simulink library "component_lib"  (R2023a)
settings: Solver=VariableStepAuto  StartTime=0.0  StopTime=10.0  RelTol=1e-3
undefined symbols (not defined in the file or in its folder): ECCV_r, par, R1234yf_ph, V_nom
libraries: base_lib x258, $bdroot x212, simulink x2, slpidlib x1
(part 7 of 7)

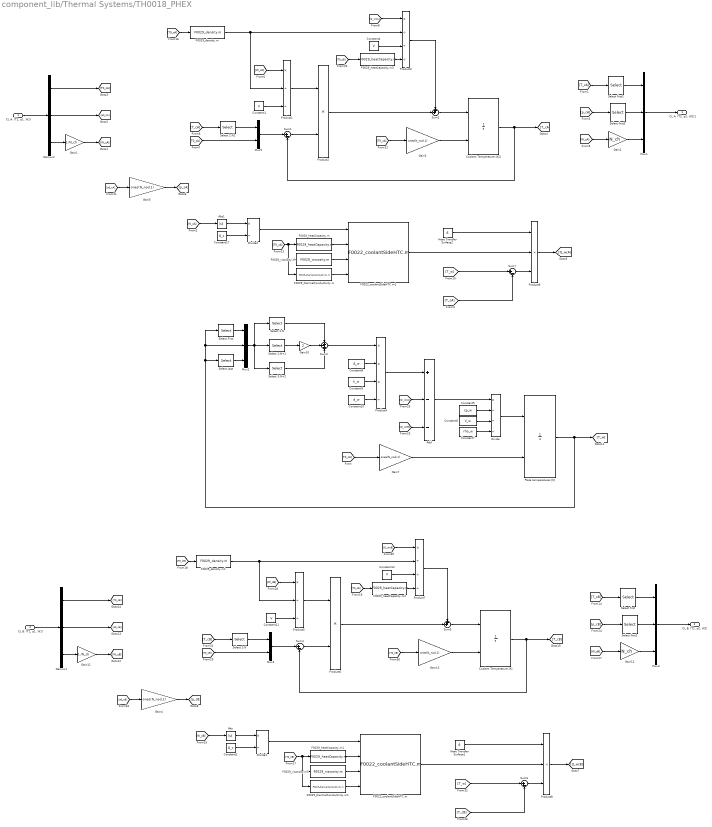
== system component_lib/Thermal Systems/TH0018_PHEX ==
  "CL A: (T1, p1, W1)" : Inport
  "CL B: (T1, p1, W1)" : Inport  Port=2
  Abs : Abs  SaturateOnIntegerOverflow=off
  Abs1 : Abs  SaturateOnIntegerOverflow=off
  Add : Sum  Inputs=+--
  Constant{1,4,11..12} (4 alike) : Constant  Value=V
  Constant10 : Constant  Value=d_w
  Constant17 : Constant  Value=A_c
  Constant2 : Constant  Value=A_c
  Constant5 : Constant  Value=cp_w
  Constant6 : Constant  Value=V_w
  Constant7 : Constant  Value=rho_w
  Constant8 : Constant  Value=A_w
  Constant9 : Constant  Value=k_w
  Coolant Temperature [K] : Integrator  InitialConditionSource=external  LimitOutput=on  LowerSaturationLimit=0
  Coolant Temperature [K]1 : Integrator  InitialConditionSource=external  LimitOutput=on  LowerSaturationLimit=0
  Demux1 : Demux  Outputs=3
  Demux2 : Demux  Outputs=3
  Divide : Product  Inputs=*///
  Divide1 : Product  Inputs=*/
  Divide2 : Product  Inputs=*/
  F0022_coolantSideHTC.m : base_lib/F0022_heatPump/F0022_coolantSideHTC.m  SystemSampleTime=-1  VariantActivationTime=update diagram  Latency=0  AutoFrameSizeCalculation=off
      settings: LibrarySourceBlock=|
      | simulink/User-Defined
      | Functions/MATLAB Function
  F0022_coolantSideHTC.m1 : base_lib/F0022_heatPump/F0022_coolantSideHTC.m  SystemSampleTime=-1  VariantActivationTime=update diagram  Latency=0  AutoFrameSizeCalculation=off
      settings: LibrarySourceBlock=|
      | simulink/User-Defined
      | Functions/MATLAB Function
  F0029_density.m : base_lib/F0029_coolantWrapper/F0029_density.m  SystemSampleTime=-1  VariantActivationTime=update diagram  Latency=0  AutoFrameSizeCalculation=off
      settings: LibrarySourceBlock=|
      | simulink/User-Defined
      | Functions/MATLAB Function
  F0029_density.m1 : base_lib/F0029_coolantWrapper/F0029_density.m  SystemSampleTime=-1  VariantActivationTime=update diagram  Latency=0  AutoFrameSizeCalculation=off
      settings: LibrarySourceBlock=|
      | simulink/User-Defined
      | Functions/MATLAB Function
  F0029_heatCapacity.m{,1..3} (4 alike) : base_lib/F0029_coolantWrapper/F0029_heatCapacity.m  SystemSampleTime=-1  VariantActivationTime=update diagram  Latency=0  AutoFrameSizeCalculation=off
      settings: LibrarySourceBlock=|
      | simulink/User-Defined
      | Functions/MATLAB Function
  F0029_thermalConductivity.m : base_lib/F0029_coolantWrapper/F0029_thermalConductivity.m  SystemSampleTime=-1  VariantActivationTime=update diagram  Latency=0  AutoFrameSizeCalculation=off
      settings: LibrarySourceBlock=|
      | simulink/User-Defined
      | Functions/MATLAB Function
  F0029_thermalConductivity.m1 : base_lib/F0029_coolantWrapper/F0029_thermalConductivity.m  SystemSampleTime=-1  VariantActivationTime=update diagram  Latency=0  AutoFrameSizeCalculation=off
      settings: LibrarySourceBlock=|
      | simulink/User-Defined
      | Functions/MATLAB Function
  F0029_viscosity.m : base_lib/F0029_coolantWrapper/F0029_viscosity.m  SystemSampleTime=-1  VariantActivationTime=update diagram  Latency=0  AutoFrameSizeCalculation=off
      settings: LibrarySourceBlock=|
      | simulink/User-Defined
      | Functions/MATLAB Function
  F0029_viscosity.m1 : base_lib/F0029_coolantWrapper/F0029_viscosity.m  SystemSampleTime=-1  VariantActivationTime=update diagram  Latency=0  AutoFrameSizeCalculation=off
      settings: LibrarySourceBlock=|
      | simulink/User-Defined
      | Functions/MATLAB Function
  Gain1 : Gain  Gain=1./N_ch
  Gain10 : Gain  Gain=2
  Gain11 : Gain  Gain=1./N_ch
  Gain12 : Gain  Gain=N_ch
  Gain{3..5,7,13} (5 alike) : Gain  Gain=ones(N_nod,1)
  Gain2 : Gain  Gain=N_ch
  Heat Transfer Surface1 : Constant  Value=A
  Heat Transfer Surface2 : Constant  Value=A
  Mux1 : Mux  Inputs=3
  Mux2 : Mux  Inputs=3
  Mux3 : Mux  Inputs=3
  Mux4 : Mux  Inputs=2
  Mux5 : Mux  Inputs=2
  Plate temperatures [K] : Integrator  InitialConditionSource=external  LimitOutput=on  LowerSaturationLimit=0
  Product1 : Product  Inputs=*//
  Product2 : Product
  Product3 : Product  Inputs=*///
  Product4 : Product  Inputs=***/
  Product5 : Product  Inputs=*//
  Product6 : Product
  Product7 : Product  Inputs=*///
  Product8 : Product  Inputs=3
  Product9 : Product  Inputs=3
  Select 1:N : Selector  InputPortWidth=N_nod+2  IndexOptions=Index vector (dialog)  Indices=[1:N_nod]  OutputSizes=1
  Select 2:N : Selector  InputPortWidth=N_nod  IndexOptions=Index vector (dialog)  Indices=[2:N_nod]  OutputSizes=1
  "Select 2:N+1 " : Selector  InputPortWidth=N_nod+2  IndexOptions=Index vector (dialog)  Indices=[2:(N_nod+1)]  OutputSizes=1
  Select 2:N1 : Selector  InputPortWidth=N_nod  IndexOptions=Index vector (dialog)  Indices=[2:N_nod]  OutputSizes=1
  Select 3:N+2 : Selector  InputPortWidth=N_nod+2  IndexOptions=Index vector (dialog)  Indices=[3:(N_nod+2)]  OutputSizes=1
  Select First : Selector  InputPortWidth=N_nod  IndexOptions=Index vector (dialog)  Indices=1  OutputSizes=1
  Select Last : Selector  InputPortWidth=N_nod  IndexOptions=Index vector (dialog)  Indices=N_nod  OutputSizes=1
  Select first{,1..3} (4 alike) : Selector  InputPortWidth=N_nod  IndexOptions=Index vector (dialog)  Indices=1  OutputSizes=1
  Sum{1,4,6..7} (4 alike) : Sum  Inputs=|+-
  Sum2 : Sum  Inputs=++|
  Sum3 : Sum  Inputs=+-+
  Sum5 : Sum  Inputs=++|
  "CL A: (T2, p2, W2)1" : Outport
  "CL B: (T2, p2, W2)" : Outport  Port=2
  wires:
  Gain7/1 -> Plate temperatures [K]/2
  Divide/1 -> Plate temperatures [K]/1
  Add/1 -> Divide/1
  Constant5/1 -> Divide/2
  Constant6/1 -> Divide/3
  Constant7/1 -> Divide/4
  [Q_wcB] -> Add/3
  Plate temperatures [K]/1 -> [T_w], Select First/1, Mux2/2, Select Last/1
  Select First/1 -> Mux2/1
  Mux2/1 -> Select 3:N+2/1, "Select 2:N+1 "/1, Select 1:N/1
  Select Last/1 -> Mux2/3
  "Select 2:N+1 "/1 -> Gain10/1
  Gain10/1 -> Sum3/2
  Select 1:N/1 -> Sum3/1
  Select 3:N+2/1 -> Sum3/3
  Sum3/1 -> Product4/1
  Constant8/1 -> Product4/2
  Constant9/1 -> Product4/3
  Constant10/1 -> Product4/4
  Product4/1 -> Add/1
  [Q_wcA] -> Add/2
  Gain11/1 -> [W_cB]
  Demux1/2 -> [p0_cB]
  "CL B: (T1, p1, W1)"/1 -> Demux1/1
  [T_cB] -> Select first/1
  Select first1/1 -> Mux3/2
  [W_cB] -> Gain12/1
  Mux3/1 -> "CL B: (T2, p2, W2)"/1
  [p_cB] -> Select first1/1
  [Q_wcB] -> Product7/1
  Mux4/1 -> Sum4/1
  Coolant Temperature [K]/1 -> [T_cB], Sum4/2
  Product7/1 -> Sum5/1
  Gain13/1 -> Coolant Temperature [K]/2
  [T_cB] -> Select 2:N/1
  Sum5/1 -> Coolant Temperature [K]/1
  Sum4/1 -> Product6/2
  F0029_density.m1/1 -> Product5/2, Product7/2
  Product5/1 -> Product6/1
  [W_cB] -> Product5/1
  Product6/1 -> Sum5/2
  Divide1/1 -> F0022_coolantSideHTC.m/1
  Product8/1 -> [Q_wcB]
  F0022_coolantSideHTC.m/1 -> Product8/2
  Sum6/1 -> Product8/3
  [T_cB] -> Sum6/2
  Gain4/1 -> [p_cB]
  [p0_cB] -> Gain4/1
  [T_w] -> Sum6/1
  Heat Transfer Surface1/1 -> Product8/1
  Constant11/1 -> Product5/3
  Constant12/1 -> Product7/3
  [T0_cB] -> Mux4/2
  Select 2:N/1 -> Mux4/1
  Gain12/1 -> Mux3/3
  Select first/1 -> Mux3/1
  Demux1/3 -> Gain11/1
  Demux1/1 -> [T0_cB]
  [T0_cA] -> Gain7/1
  [T0_cB] -> Gain13/1
  Abs/1 -> Divide1/1
  Constant2/1 -> Divide1/2
  [W_cB] -> Abs/1
  [T_cA] -> Sum7/2
  Gain2/1 -> Mux1/3
  Select 2:N1/1 -> Mux5/1
  Select first2/1 -> Mux1/1
  Demux2/2 -> [p0_cA]
  Divide2/1 -> F0022_coolantSideHTC.m1/1
  [T_cA] -> Select first2/1
  Constant1/1 -> Product1/3
  [W_cA] -> Product1/1
  Gain5/1 -> [p_cA]
  Sum7/1 -> Product9/3
  Demux2/3 -> Gain1/1
  [Q_wcA] -> Product3/1
  F0022_coolantSideHTC.m1/1 -> Product9/2
  [T0_cA] -> Mux5/2
  [W_cA] -> Abs1/1
  Constant17/1 -> Divide2/2
  Sum2/1 -> Coolant Temperature [K]1/1
  F0029_density.m/1 -> Product3/2, Product1/2
  Demux2/1 -> [T0_cA]
  [T0_cA] -> Gain3/1
  Gain1/1 -> [W_cA]
  Sum1/1 -> Product2/2
  [T_cA] -> Select 2:N1/1
  Product3/1 -> Sum2/1
  Gain3/1 -> Coolant Temperature [K]1/2
  [p_cA] -> Select first3/1
  Mux5/1 -> Sum1/1
  Coolant Temperature [K]1/1 -> [T_cA], Sum1/2
  Constant4/1 -> Product3/3
  Product2/1 -> Sum2/2
  Product9/1 -> [Q_wcA]
  [T_w] -> Sum7/1
  Mux1/1 -> "CL A: (T2, p2, W2)1"/1
  Product1/1 -> Product2/1
  Select first3/1 -> Mux1/2
  [p0_cA] -> Gain5/1
  "CL A: (T1, p1, W1)"/1 -> Demux2/1
  Heat Transfer Surface2/1 -> Product9/1
  [W_cA] -> Gain2/1
  Abs1/1 -> Divide2/1
  F0029_heatCapacity.m/1 -> F0022_coolantSideHTC.m1/2
  F0029_viscosity.m/1 -> F0022_coolantSideHTC.m1/3
  F0029_thermalConductivity.m/1 -> F0022_coolantSideHTC.m1/4
  [T0_cA] -> F0029_thermalConductivity.m/1, F0029_viscosity.m/1, F0029_heatCapacity.m/1
  F0029_heatCapacity.m1/1 -> F0022_coolantSideHTC.m/2
  [T0_cB] -> F0029_thermalConductivity.m1/1, F0029_viscosity.m1/1, F0029_heatCapacity.m1/1
  F0029_viscosity.m1/1 -> F0022_coolantSideHTC.m/3
  F0029_thermalConductivity.m1/1 -> F0022_coolantSideHTC.m/4
  [T0_cA] -> F0029_density.m/1
  [T0_cB] -> F0029_density.m1/1
  F0029_heatCapacity.m2/1 -> Product7/4
  [T0_cB] -> F0029_heatCapacity.m2/1
  F0029_heatCapacity.m3/1 -> Product3/4
  [T0_cB] -> F0029_heatCapacity.m3/1

== system component_lib/Thermal Systems/TH0019_airTotalHeatTransfer ==
  Q [J/s] : Inport
  AIR: (T1,p1,W1) : Inport  Port=2
  Constant : Constant  Value=par.cp_air
  Demux : Demux  Outputs=3
  Mux : Mux  Inputs=3
  Product : Product  Inputs=*//
  Saturation : Saturate  UpperLimit=T_max  LowerLimit=T_min
  Saturation1 : Saturate  UpperLimit=inf  LowerLimit=0.001
  Sum : Sum  Inputs=++|
  AIR: (T2,p2,W2) : Outport
  wires:
  AIR: (T1,p1,W1)/1 -> Demux/1
  Mux/1 -> AIR: (T2,p2,W2)/1
  Demux/3 -> Mux/3, Saturation1/1
  Demux/2 -> Mux/2
  Q [J/s]/1 -> Product/1
  Constant/1 -> Product/3
  Demux/1 -> Sum/2
  Product/1 -> Sum/1
  Sum/1 -> Saturation/1
  Saturation/1 -> Mux/1
  Saturation1/1 -> Product/2

== system component_lib/Thermal Systems/TH0020_cm100hp ==
  V_sup [V] : Inport
  V_ctrl [V] : Inport  Port=2
  CL: (T1,p1,W1) : Inport  Port=3
  Constant5 : Constant  Value=27.5
  Demux : Demux  Outputs=3
  Divide : Product  Inputs=/*
  Divide1 : Product  Inputs=*/
  F0023_current.m : base_lib/F0023_epirocWaterPump/F0023_current.m  SystemSampleTime=-1  VariantActivationTime=update diagram  Latency=0  AutoFrameSizeCalculation=off
      settings: LibrarySourceBlock=|
      | simulink/User-Defined
      | Functions/MATLAB Function
  F0023_pressure.m : base_lib/F0023_epirocWaterPump/F0023_pressure.m  SystemSampleTime=-1  VariantActivationTime=update diagram  Latency=0  AutoFrameSizeCalculation=off
      settings: LibrarySourceBlock=|
      | simulink/User-Defined
      | Functions/MATLAB Function
  F0023_speed.m : base_lib/F0023_epirocWaterPump/F0023_speed.m  SystemSampleTime=-1  VariantActivationTime=update diagram  Latency=0  AutoFrameSizeCalculation=off
      settings: LibrarySourceBlock=|
      | simulink/User-Defined
      | Functions/MATLAB Function
  Gain : Gain  Gain=1e5
  Gain1 : Gain
  Integrator Limited : Integrator  InitialConditionSource=external  LimitOutput=on  UpperSaturationLimit=10  LowerSaturationLimit=0
  Mux : Mux  Inputs=3
  Product1 : Product  Inputs=3
  Sum : Sum  Inputs=|++
  Sum1 : Sum  Inputs=-|+
  Terminator : Terminator
  I [A] : Outport
  CL: (T2,p2,W2) : Outport  Port=2
  wires:
  CL: (T1,p1,W1)/1 -> Demux/1
  Mux/1 -> CL: (T2,p2,W2)/1
  Integrator Limited/1 -> F0023_speed.m/2, F0023_current.m/2, Sum1/1, F0023_pressure.m/2
  Demux/2 -> Sum/1
  Sum/1 -> Mux/2
  Demux/3 -> [q], F0023_speed.m/1, F0023_current.m/1, F0023_pressure.m/1, Mux/3
  Demux/1 -> Mux/1
  F0023_pressure.m/1 -> Gain/1
  Sum1/1 -> Gain1/1
  V_ctrl [V]/1 -> Sum1/2, Integrator Limited/2
  Gain1/1 -> Integrator Limited/1
  V_sup [V]/1 -> Divide1/2, [V_sup]
  Divide1/1 -> I [A]/1
  [V_sup] -> Divide/1, Product1/1
  F0023_current.m/1 -> Product1/3
  Divide/1 -> Product1/2
  Constant5/1 -> Divide/2
  Product1/1 -> Divide1/1
  F0023_speed.m/1 -> Terminator/1
  Gain/1 -> Sum/2

== system component_lib/Thermal Systems/TH0020_staticPressureDrop ==
  CL: (T1,p1,W1) : Inport
  Constant : Constant  Value=dp
  Demux : Demux  Outputs=3
  Mux : Mux  Inputs=3
  Sum : Sum  Inputs=|+-
  CL: (T2,p2,W2) : Outport
  wires:
  CL: (T1,p1,W1)/1 -> Demux/1
  Mux/1 -> CL: (T2,p2,W2)/1
  Demux/2 -> Sum/1
  Sum/1 -> Mux/2
  Demux/3 -> Mux/3
  Demux/1 -> Mux/1
  Constant/1 -> Sum/2

== system component_lib/Thermal Systems/TH0021_tank ==
  p [Pa] : Inport
  CL: (T1,p1,W1) : Inport  Port=2
  Constant2 : Constant  Value=T0
  Demux1 : Demux  Outputs=3
  Gain : Gain  Gain=1e-3
  Gain1 : Gain  Gain=1e-1
  Integrator : Integrator  InitialCondition=1  LimitOutput=on  LowerSaturationLimit=0
  Integrator2 : Integrator  InitialConditionSource=external  InitialCondition=293  LimitOutput=on  LowerSaturationLimit=1e-3
  Mux1 : Mux  Inputs=3
  Sum : Sum  Inputs=-+|
  Sum2 : Sum  Inputs=|+-
  W [kg/s] : Outport
  CL: (T2,p2,W2) : Outport  Port=2
  wires:
  Demux1/1 -> Sum2/1
  Constant2/1 -> Integrator2/2
  Integrator2/1 -> [T], Mux1/1
  Mux1/1 -> CL: (T2,p2,W2)/1
  Gain1/1 -> Integrator2/1
  CL: (T1,p1,W1)/1 -> Demux1/1
  p [Pa]/1 -> Sum/1, Mux1/2
  Demux1/2 -> [p1]
  [T] -> Sum2/2
  Gain/1 -> Integrator/1
  [p1] -> Sum/2
  Integrator/1 -> W [kg/s]/1, Mux1/3
  Sum/1 -> Gain/1
  Sum2/1 -> Gain1/1

== system component_lib/Thermal Systems/TH0022_restriction ==
  CL: (T1,p1,W1) : Inport
  Demux : Demux  Outputs=3
  F0017_restriction.m : base_lib/F0017_channelCooling/F0017_restriction.m  SystemSampleTime=-1  VariantActivationTime=update diagram  Latency=0  AutoFrameSizeCalculation=off
      settings: LibrarySourceBlock=|
      | simulink/User-Defined
      | Functions/MATLAB Function
  F0029_density.m : base_lib/F0029_coolantWrapper/F0029_density.m  SystemSampleTime=-1  VariantActivationTime=update diagram  Latency=0  AutoFrameSizeCalculation=off
      settings: LibrarySourceBlock=|
      | simulink/User-Defined
      | Functions/MATLAB Function
  Mux : Mux  Inputs=3
  Sum : Sum  Inputs=|+-
  CL: (T2,p2,W2) : Outport
  wires:
  CL: (T1,p1,W1)/1 -> Demux/1
  Mux/1 -> CL: (T2,p2,W2)/1
  Demux/3 -> Mux/3, F0017_restriction.m/1
  Demux/2 -> Sum/1
  Sum/1 -> Mux/2
  F0017_restriction.m/1 -> Sum/2
  F0029_density.m/1 -> F0017_restriction.m/2
  Demux/1 -> F0029_density.m/1, Mux/1

== system component_lib/Thermal Systems/TH0023_WP120 ==
  V_sup [V] : Inport
  n [rpm] : Inport  Port=2
  CL: (T1,p1,W1) : Inport  Port=3
  Demux : Demux  Outputs=3
  Divide : Product  Inputs=*/
  F0024_powerWP120.m : base_lib/F0024_WPpumps/F0024_powerWP120.m  SystemSampleTime=-1  VariantActivationTime=update diagram  Latency=0  AutoFrameSizeCalculation=off
      settings: LibrarySourceBlock=|
      | simulink/User-Defined
      | Functions/MATLAB Function
  F0024_pressureWP120.m : base_lib/F0024_WPpumps/F0024_pressureWP120.m  SystemSampleTime=-1  VariantActivationTime=update diagram  Latency=0  AutoFrameSizeCalculation=off
      settings: LibrarySourceBlock=|
      | simulink/User-Defined
      | Functions/MATLAB Function
  Gain1 : Gain
  Integrator Limited : Integrator  InitialConditionSource=external  LimitOutput=on  UpperSaturationLimit=6000  LowerSaturationLimit=0
  Mux : Mux  Inputs=3
  Sum : Sum  Inputs=|++
  Sum1 : Sum  Inputs=-|+
  I [A] : Outport
  CL: (T2,p2,W2) : Outport  Port=2
  wires:
  F0024_pressureWP120.m/1 -> Sum/2
  F0024_powerWP120.m/1 -> Divide/1
  Gain1/1 -> Integrator Limited/1
  n [rpm]/1 -> Integrator Limited/2, Sum1/2
  Sum1/1 -> Gain1/1
  Demux/1 -> Mux/1
  Demux/3 -> Mux/3, F0024_powerWP120.m/1, F0024_pressureWP120.m/1, [q]
  Sum/1 -> Mux/2
  Demux/2 -> Sum/1
  Integrator Limited/1 -> F0024_powerWP120.m/2, F0024_pressureWP120.m/2, Sum1/1
  Mux/1 -> CL: (T2,p2,W2)/1
  CL: (T1,p1,W1)/1 -> Demux/1
  Divide/1 -> I [A]/1
  V_sup [V]/1 -> Divide/2

== system component_lib/Thermal Systems/TH0024_WP150 ==
  V_sup [V] : Inport
  n [rpm] : Inport  Port=2
  CL: (T1,p1,W1) : Inport  Port=3
  Demux : Demux  Outputs=3
  Divide : Product  Inputs=*/
  F0024_powerWP150.m : base_lib/F0024_WPpumps/F0024_powerWP150.m  SystemSampleTime=-1  VariantActivationTime=update diagram  Latency=0  AutoFrameSizeCalculation=off
      settings: LibrarySourceBlock=|
      | simulink/User-Defined
      | Functions/MATLAB Function
  F0024_pressureWP150.m : base_lib/F0024_WPpumps/F0024_pressureWP150.m  SystemSampleTime=-1  VariantActivationTime=update diagram  Latency=0  AutoFrameSizeCalculation=off
      settings: LibrarySourceBlock=|
      | simulink/User-Defined
      | Functions/MATLAB Function
  Gain : Gain  Gain=1/n
  Gain1 : Gain
  Gain2 : Gain  Gain=n
  Gain3 : Gain  Gain=n
  Integrator Limited : Integrator  InitialConditionSource=external  LimitOutput=on  UpperSaturationLimit=4500  LowerSaturationLimit=0
  Mux : Mux  Inputs=3
  Sum : Sum  Inputs=|++
  Sum1 : Sum  Inputs=-|+
  I [A] : Outport
  CL: (T2,p2,W2) : Outport  Port=2
  wires:
  F0024_pressureWP150.m/1 -> Sum/2
  F0024_powerWP150.m/1 -> Divide/1
  Gain1/1 -> Integrator Limited/1
  n [rpm]/1 -> Integrator Limited/2, Sum1/2
  Sum1/1 -> Gain1/1
  Demux/1 -> Mux/1
  Demux/3 -> Gain/1
  Sum/1 -> Mux/2
  Demux/2 -> Sum/1
  Integrator Limited/1 -> F0024_powerWP150.m/2, F0024_pressureWP150.m/2, Sum1/1
  Mux/1 -> CL: (T2,p2,W2)/1
  CL: (T1,p1,W1)/1 -> Demux/1
  Divide/1 -> Gain3/1
  V_sup [V]/1 -> Divide/2
  Gain/1 -> Gain2/1, F0024_powerWP150.m/1, F0024_pressureWP150.m/1, [q]
  Gain2/1 -> Mux/3
  Gain3/1 -> I [A]/1

== system component_lib/Thermal Systems/TH0025_VA164A ==
  V_sup [V] : Inport
  n [rpm] : Inport  Port=2
  AIR: (T1,p1,W1) : Inport  Port=3
  Demux : Demux  Outputs=3
  Divide : Product  Inputs=*/
  F0025_powerVA164A.m : base_lib/F0025_spalFans/F0025_powerVA164A.m  SystemSampleTime=-1  VariantActivationTime=update diagram  Latency=0  AutoFrameSizeCalculation=off
      settings: LibrarySourceBlock=|
      | simulink/User-Defined
      | Functions/MATLAB Function
  F0025_pressureVA164A.m : base_lib/F0025_spalFans/F0025_pressureVA164A.m  SystemSampleTime=-1  VariantActivationTime=update diagram  Latency=0  AutoFrameSizeCalculation=off
      settings: LibrarySourceBlock=|
      | simulink/User-Defined
      | Functions/MATLAB Function
  Gain : Gain  Gain=1/n
  Gain1 : Gain
  Gain2 : Gain  Gain=n
  Integrator Limited : Integrator  InitialConditionSource=external  LimitOutput=on  UpperSaturationLimit=3000  LowerSaturationLimit=0
  Mux : Mux  Inputs=3
  Sum : Sum  Inputs=|++
  Sum1 : Sum  Inputs=-|+
  I [A] : Outport
  AIR: (T2,p2,W2) : Outport  Port=2
  wires:
  F0025_pressureVA164A.m/1 -> Sum/2
  F0025_powerVA164A.m/1 -> Gain2/1
  Gain1/1 -> Integrator Limited/1
  n [rpm]/1 -> Integrator Limited/2, Sum1/2
  Sum1/1 -> Gain1/1
  Demux/1 -> Mux/1
  Demux/3 -> Mux/3, Gain/1, [q]
  Sum/1 -> Mux/2
  Demux/2 -> Sum/1
  Integrator Limited/1 -> F0025_pressureVA164A.m/2, F0025_powerVA164A.m/2, Sum1/1
  Mux/1 -> AIR: (T2,p2,W2)/1
  AIR: (T1,p1,W1)/1 -> Demux/1
  Divide/1 -> I [A]/1
  V_sup [V]/1 -> Divide/2
  Gain/1 -> F0025_pressureVA164A.m/1, F0025_powerVA164A.m/1
  Gain2/1 -> Divide/1

== system component_lib/Thermal Systems/TH0026_airVolume ==
  dQ [J/s] : Inport
  AIR: (T1,p1,W1) : Inport  Port=2
  Constant : Constant  Value=par.cp_air
  Constant1 : Constant  Value=T0
  Constant2 : Constant  Value=par.rho_air
  Constant3 : Constant  Value=V
  Demux1 : Demux  Outputs=3
  Divide : Product  Inputs=*/
  Divide1 : Product  Inputs=*/
  Gain : Gain  Gain=1e3
  Gain1 : Gain  Gain=1e3
  Integrator : Integrator  InitialConditionSource=external
  Integrator1 : Integrator  InitialCondition=1e5
  Integrator2 : Integrator
  Mux1 : Mux  Inputs=3
  Product : Product
  Product2 : Product
  Product3 : Product
  Sum : Sum  Inputs=++|
  Sum1 : Sum  Inputs=+|-
  Sum2 : Sum  Inputs=|+-
  Sum3 : Sum  Inputs=|+-
  T [K] : Outport
  AIR: (T2,p2,W2) : Outport  Port=2
  wires:
  Mux1/1 -> AIR: (T2,p2,W2)/1
  AIR: (T1,p1,W1)/1 -> Demux1/1
  Demux1/2 -> Sum2/1
  Constant1/1 -> Integrator/2
  dQ [J/s]/1 -> Divide/1
  Constant/1 -> Divide/2
  Divide/1 -> Sum/1
  Constant3/1 -> Product/1
  Constant2/1 -> Product/2
  Sum/1 -> Divide1/1
  Divide1/1 -> Integrator/1
  Product/1 -> Divide1/2
  Integrator/1 -> T [K]/1, Product3/1, Mux1/1
  Sum1/1 -> Sum/2
  Demux1/1 -> Product2/1
  Product2/1 -> Sum1/1
  Product3/1 -> Sum1/2
  Sum2/1 -> Gain/1
  Gain/1 -> Integrator1/1
  Integrator1/1 -> Mux1/2, Sum2/2
  Gain1/1 -> Integrator2/1
  Sum3/1 -> Gain1/1
  Demux1/3 -> Product2/2, Sum3/1
  Integrator2/1 -> Sum3/2, Product3/2, Mux1/3

== system component_lib/Thermal Systems/TH0027_hvacFlap ==
  open [-] : Inport
  AIR: (T1,p1,W1) : Inport  Port=2
  Demux1 : Demux  Outputs=3
  F0014_variableAreaPressureDrop.m : base_lib/F0014_titanXradiator/F0014_variableAreaPressureDrop.m  SystemSampleTime=-1  VariantActivationTime=update diagram  Latency=0  AutoFrameSizeCalculation=off
      settings: LibrarySourceBlock=|
      | simulink/User-Defined
      | Functions/MATLAB Function
  Mux1 : Mux  Inputs=3
  Saturation : Saturate  UpperLimit=1  LowerLimit=0
  Sum : Sum  Inputs=-+|
  AIR: (T2,p2,W2) : Outport
  wires:
  Mux1/1 -> AIR: (T2,p2,W2)/1
  AIR: (T1,p1,W1)/1 -> Demux1/1
  Demux1/3 -> Mux1/3, F0014_variableAreaPressureDrop.m/3
  Demux1/1 -> Mux1/1, F0014_variableAreaPressureDrop.m/1
  F0014_variableAreaPressureDrop.m/1 -> Sum/1
  Sum/1 -> Mux1/2
  Demux1/2 -> F0014_variableAreaPressureDrop.m/2, Sum/2
  open [-]/1 -> Saturation/1
  Saturation/1 -> F0014_variableAreaPressureDrop.m/4

== system component_lib/Thermal Systems/TH0028_VA195 ==
  V_sup [V] : Inport
  n [rpm] : Inport  Port=2
  AIR: (T1,p1,W1) : Inport  Port=3
  Demux : Demux  Outputs=3
  Divide : Product  Inputs=*/
  F0025_powerVA195.m : base_lib/F0025_spalFans/F0025_powerVA195.m  SystemSampleTime=-1  VariantActivationTime=update diagram  Latency=0  AutoFrameSizeCalculation=off
      settings: LibrarySourceBlock=|
      | simulink/User-Defined
      | Functions/MATLAB Function
  F0025_pressureVA195.m : base_lib/F0025_spalFans/F0025_pressureVA195.m  SystemSampleTime=-1  VariantActivationTime=update diagram  Latency=0  AutoFrameSizeCalculation=off
      settings: LibrarySourceBlock=|
      | simulink/User-Defined
      | Functions/MATLAB Function
  Gain : Gain  Gain=1/n
  Gain1 : Gain
  Gain2 : Gain  Gain=n
  Integrator Limited : Integrator  InitialConditionSource=external  LimitOutput=on  UpperSaturationLimit=5000  LowerSaturationLimit=0
  Mux : Mux  Inputs=3
  Sum : Sum  Inputs=|++
  Sum1 : Sum  Inputs=-|+
  I [A] : Outport
  AIR: (T2,p2,W2) : Outport  Port=2
  wires:
  F0025_pressureVA195.m/1 -> Sum/2
  F0025_powerVA195.m/1 -> Gain2/1
  Gain1/1 -> Integrator Limited/1
  n [rpm]/1 -> Integrator Limited/2, Sum1/2
  Sum1/1 -> Gain1/1
  Demux/1 -> Mux/1
  Demux/3 -> Gain/1, Mux/3
  Sum/1 -> Mux/2
  Demux/2 -> Sum/1
  Integrator Limited/1 -> F0025_powerVA195.m/2, F0025_pressureVA195.m/2, Sum1/1
  Mux/1 -> AIR: (T2,p2,W2)/1
  AIR: (T1,p1,W1)/1 -> Demux/1
  Divide/1 -> I [A]/1
  V_sup [V]/1 -> Divide/2
  Gain/1 -> F0025_powerVA195.m/1, F0025_pressureVA195.m/1
  Gain2/1 -> Divide/1

== system component_lib/Thermal Systems/TH0029_cabinConvection ==
  v [m/s] : Inport
  T_amb [K] : Inport  Port=2
  T_cabin [K] : Inport  Port=3
  Constant : Constant  Value=A
  F0017_vehicleSurfaceHTC.m : base_lib/F0017_channelCooling/F0017_vehicleSurfaceHTC.m  SystemSampleTime=-1  VariantActivationTime=update diagram  Latency=0  AutoFrameSizeCalculation=off
      settings: LibrarySourceBlock=|
      | simulink/User-Defined
      | Functions/MATLAB Function
  Product : Product  Inputs=3
  Sum : Sum  Inputs=|+-
  Q [J/s] : Outport
  wires:
  v [m/s]/1 -> F0017_vehicleSurfaceHTC.m/1
  T_amb [K]/1 -> Sum/1
  T_cabin [K]/1 -> Sum/2
  Sum/1 -> Product/1
  F0017_vehicleSurfaceHTC.m/1 -> Product/3
  Constant/1 -> Product/2
  Product/1 -> Q [J/s]/1

== system component_lib/Thermal Systems/TH0030_batteryPackConvection ==
  T_amb [K] : Inport
  T_bat [K] : Inport  Port=2
  Constant : Constant  Value=A
  Constant1 : Constant  Value=h
  Product : Product  Inputs=3
  Sum : Sum  Inputs=|+-
  Q [J/s] : Outport
  wires:
  T_amb [K]/1 -> Sum/1
  T_bat [K]/1 -> Sum/2
  Sum/1 -> Product/1
  Constant/1 -> Product/2
  Product/1 -> Q [J/s]/1
  Constant1/1 -> Product/3

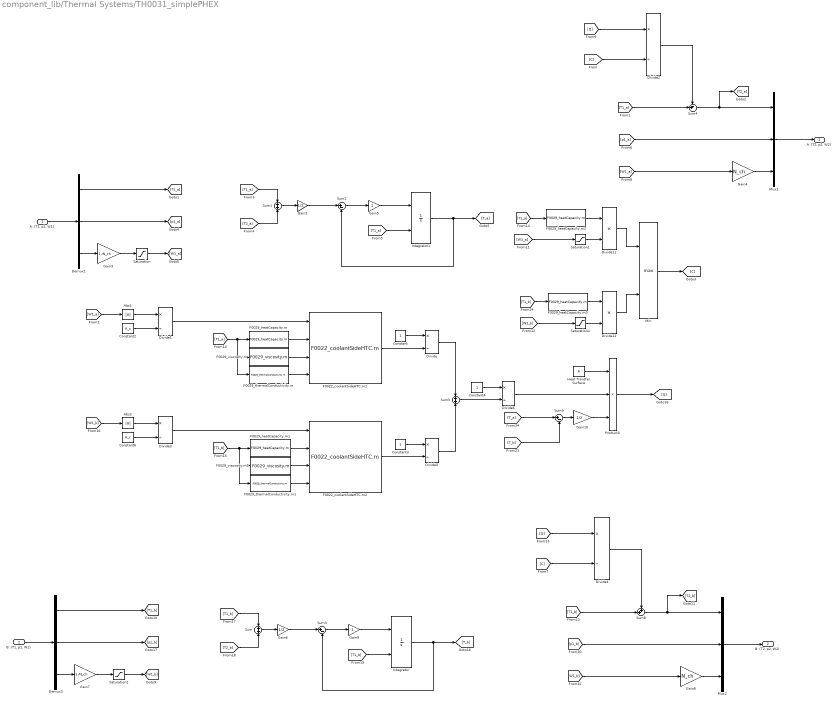
== system component_lib/Thermal Systems/TH0031_simplePHEX ==
  "A: (T1, p1, W1)" : Inport
  "B: (T1, p1, W1)" : Inport  Port=2
  Abs1 : Abs  SaturateOnIntegerOverflow=off
  Abs2 : Abs  SaturateOnIntegerOverflow=off
  Constant : Constant
  Constant2 : Constant  Value=A_c
  Constant3 : Constant
  Constant4 : Constant
  Constant6 : Constant  Value=A_c
  Demux1 : Demux  Outputs=3
  Demux3 : Demux  Outputs=3
  Divide{,1..6} (7 alike) : Product  Inputs=*/
  Divide11 : Product  Inputs=**
  Divide12 : Product  Inputs=**
  F0022_coolantSideHTC.m1 : base_lib/F0022_heatPump/F0022_coolantSideHTC.m  SystemSampleTime=-1  VariantActivationTime=update diagram  Latency=0  AutoFrameSizeCalculation=off
      settings: LibrarySourceBlock=|
      | simulink/User-Defined
      | Functions/MATLAB Function
  F0022_coolantSideHTC.m2 : base_lib/F0022_heatPump/F0022_coolantSideHTC.m  SystemSampleTime=-1  VariantActivationTime=update diagram  Latency=0  AutoFrameSizeCalculation=off
      settings: LibrarySourceBlock=|
      | simulink/User-Defined
      | Functions/MATLAB Function
  F0029_heatCapacity.m{,1..3} (4 alike) : base_lib/F0029_coolantWrapper/F0029_heatCapacity.m  SystemSampleTime=-1  VariantActivationTime=update diagram  Latency=0  AutoFrameSizeCalculation=off
      settings: LibrarySourceBlock=|
      | simulink/User-Defined
      | Functions/MATLAB Function
  F0029_thermalConductivity.m : base_lib/F0029_coolantWrapper/F0029_thermalConductivity.m  SystemSampleTime=-1  VariantActivationTime=update diagram  Latency=0  AutoFrameSizeCalculation=off
      settings: LibrarySourceBlock=|
      | simulink/User-Defined
      | Functions/MATLAB Function
  F0029_thermalConductivity.m1 : base_lib/F0029_coolantWrapper/F0029_thermalConductivity.m  SystemSampleTime=-1  VariantActivationTime=update diagram  Latency=0  AutoFrameSizeCalculation=off
      settings: LibrarySourceBlock=|
      | simulink/User-Defined
      | Functions/MATLAB Function
  F0029_viscosity.m : base_lib/F0029_coolantWrapper/F0029_viscosity.m  SystemSampleTime=-1  VariantActivationTime=update diagram  Latency=0  AutoFrameSizeCalculation=off
      settings: LibrarySourceBlock=|
      | simulink/User-Defined
      | Functions/MATLAB Function
  F0029_viscosity.m1 : base_lib/F0029_coolantWrapper/F0029_viscosity.m  SystemSampleTime=-1  VariantActivationTime=update diagram  Latency=0  AutoFrameSizeCalculation=off
      settings: LibrarySourceBlock=|
      | simulink/User-Defined
      | Functions/MATLAB Function
  Gain10 : Gain  Gain=1/2
  Gain2 : Gain  Gain=1/2
  Gain3 : Gain  Gain=1./N_ch
  Gain4 : Gain  Gain=N_ch
  Gain5 : Gain
  Gain6 : Gain  Gain=1/2
  Gain7 : Gain  Gain=1./N_ch
  Gain8 : Gain  Gain=N_ch
  Gain9 : Gain
  Heat Transfer Surface : Constant  Value=A
  Integrator : Integrator  InitialConditionSource=external  LimitOutput=on  UpperSaturationLimit=273+100  LowerSaturationLimit=273-40
  Integrator1 : Integrator  InitialConditionSource=external  LimitOutput=on  UpperSaturationLimit=273+100  LowerSaturationLimit=273-40
  Min : MinMax  Function=max  Inputs=2
  Mux1 : Mux  Inputs=3
  Mux2 : Mux  Inputs=3
  Product4 : Product  Inputs=3
  Saturation : Saturate  UpperLimit=inf  LowerLimit=1e-5
  Saturation1 : Saturate  UpperLimit=inf  LowerLimit=0.0001
  Saturation2 : Saturate  UpperLimit=inf  LowerLimit=1e-5
  Saturation4 : Saturate  UpperLimit=inf  LowerLimit=0.0001
  Sum : Sum  Inputs=+|+
  Sum1 : Sum  Inputs=+|+
  Sum2 : Sum  Inputs=|+-
  Sum3 : Sum  Inputs=|+-
  Sum4 : Sum  Inputs=-+|
  Sum5 : Sum  Inputs=+|+
  Sum8 : Sum  Inputs=++|
  Sum9 : Sum  Inputs=|+-
  "A: (T2, p2, W2)" : Outport
  "B: (T2, p2, W2)" : Outport  Port=2
  wires:
  [T2_b] -> Sum/2
  [W1_b] -> Gain8/1
  [T1_b] -> Integrator/2
  Gain10/1 -> Product4/3
  Constant6/1 -> Divide3/2
  [T1_b] -> Sum/1
  Gain6/1 -> Sum3/1
  Gain9/1 -> Integrator/1
  Heat Transfer Surface/1 -> Product4/1
  Demux3/2 -> [p1_b]
  [T1_b] -> Sum8/2
  [Q] -> Divide4/1
  Integrator/1 -> [T_b], Sum3/2
  Divide3/1 -> F0022_coolantSideHTC.m2/1
  Sum9/1 -> Gain10/1
  [T_a] -> Sum9/1
  Sum8/1 -> Mux2/1, [T2_b]
  Demux3/1 -> [T1_b]
  Sum3/1 -> Gain9/1
  [T_b] -> Sum9/2
  [W1_b] -> Abs2/1
  Mux2/1 -> "B: (T2, p2, W2)"/1
  Demux3/3 -> Gain7/1
  Divide4/1 -> Sum8/1
  [p1_b] -> Mux2/2
  Gain8/1 -> Mux2/3
  Sum/1 -> Gain6/1
  Abs2/1 -> Divide3/1
  "B: (T1, p1, W1)"/1 -> Demux3/1
  Divide2/1 -> Sum4/1
  [p1_a] -> Mux1/2
  [T1_a] -> Sum1/1
  Abs1/1 -> Divide1/1
  Divide1/1 -> F0022_coolantSideHTC.m1/1
  Gain2/1 -> Sum2/1
  [T1_a] -> Sum4/2
  "A: (T1, p1, W1)"/1 -> Demux1/1
  Sum2/1 -> Gain5/1
  Demux1/1 -> [T1_a]
  [T1_a] -> Integrator1/2
  Mux1/1 -> "A: (T2, p2, W2)"/1
  [W1_a] -> Gain4/1
  Constant2/1 -> Divide1/2
  Gain3/1 -> Saturation/1
  [Q] -> Divide2/1
  Demux1/2 -> [p1_a]
  Integrator1/1 -> [T_a], Sum2/2
  Sum4/1 -> Mux1/1, [T2_a]
  [T2_a] -> Sum1/2
  [W1_a] -> Abs1/1
  Sum1/1 -> Gain2/1
  Demux1/3 -> Gain3/1
  Gain4/1 -> Mux1/3
  Gain5/1 -> Integrator1/1
  Constant/1 -> Divide/1
  F0022_coolantSideHTC.m1/1 -> Divide/2
  F0022_coolantSideHTC.m2/1 -> Divide5/2
  Constant3/1 -> Divide5/1
  Divide/1 -> Sum5/1
  Divide5/1 -> Sum5/2
  Constant4/1 -> Divide6/1
  Sum5/1 -> Divide6/2
  Divide6/1 -> Product4/2
  [C] -> Divide2/2
  Product4/1 -> [Q]
  [W1_a] -> Saturation1/1
  Saturation1/1 -> Divide11/2
  [W1_b] -> Saturation4/1
  Saturation4/1 -> Divide12/2
  Divide11/1 -> Min/1
  Divide12/1 -> Min/2
  Min/1 -> [C]
  [C] -> Divide4/2
  Saturation/1 -> [W1_a]
  Gain7/1 -> Saturation2/1
  Saturation2/1 -> [W1_b]
  F0029_viscosity.m/1 -> F0022_coolantSideHTC.m1/3
  F0029_thermalConductivity.m/1 -> F0022_coolantSideHTC.m1/4
  F0029_heatCapacity.m/1 -> F0022_coolantSideHTC.m1/2
  [T1_a] -> F0029_thermalConductivity.m/1, F0029_viscosity.m/1, F0029_heatCapacity.m/1
  F0029_heatCapacity.m1/1 -> F0022_coolantSideHTC.m2/2
  F0029_thermalConductivity.m1/1 -> F0022_coolantSideHTC.m2/4
  [T1_b] -> F0029_thermalConductivity.m1/1, F0029_viscosity.m1/1, F0029_heatCapacity.m1/1
  F0029_viscosity.m1/1 -> F0022_coolantSideHTC.m2/3
  [T1_a] -> F0029_heatCapacity.m2/1
  F0029_heatCapacity.m2/1 -> Divide11/1
  [T1_b] -> F0029_heatCapacity.m3/1
  F0029_heatCapacity.m3/1 -> Divide12/1

== system component_lib/Thermal Systems/TH0032_VA113 ==
  V_sup [V] : Inport
  n [rpm] : Inport  Port=2
  AIR: (T1,p1,W1) : Inport  Port=3
  Demux : Demux  Outputs=3
  Divide : Product  Inputs=*/
  F0025_powerVA113.m : base_lib/F0025_spalFans/F0025_powerVA113.m  SystemSampleTime=-1  VariantActivationTime=update diagram  Latency=0  AutoFrameSizeCalculation=off
      settings: LibrarySourceBlock=|
      | simulink/User-Defined
      | Functions/MATLAB Function
  F0025_pressureVA113.m : base_lib/F0025_spalFans/F0025_pressureVA113.m  SystemSampleTime=-1  VariantActivationTime=update diagram  Latency=0  AutoFrameSizeCalculation=off
      settings: LibrarySourceBlock=|
      | simulink/User-Defined
      | Functions/MATLAB Function
  Gain : Gain  Gain=1/n
  Gain1 : Gain  Gain=10
  Gain2 : Gain  Gain=n
  Integrator Limited : Integrator  InitialConditionSource=external  LimitOutput=on  UpperSaturationLimit=4750  LowerSaturationLimit=0
  Mux : Mux  Inputs=3
  Sum : Sum  Inputs=|++
  Sum1 : Sum  Inputs=-|+
  I [A] : Outport
  AIR: (T2,p2,W2) : Outport  Port=2
  wires:
  F0025_pressureVA113.m/1 -> Sum/2
  F0025_powerVA113.m/1 -> Gain2/1
  Gain1/1 -> Integrator Limited/1
  n [rpm]/1 -> Integrator Limited/2, Sum1/2
  Sum1/1 -> Gain1/1
  Demux/1 -> Mux/1
  Demux/3 -> Mux/3, Gain/1, [q]
  Sum/1 -> Mux/2
  Demux/2 -> Sum/1
  Integrator Limited/1 -> F0025_powerVA113.m/2, F0025_pressureVA113.m/2, Sum1/1
  Mux/1 -> AIR: (T2,p2,W2)/1
  AIR: (T1,p1,W1)/1 -> Demux/1
  Divide/1 -> I [A]/1
  V_sup [V]/1 -> Divide/2
  Gain/1 -> F0025_powerVA113.m/1, F0025_pressureVA113.m/1
  Gain2/1 -> Divide/1

== system component_lib/Thermal Systems/RF0007_PHEX/Heat Tranfer Coefficient - Refrigerant Side ==
  W_r [kg/s] : Inport
  x_r [-] : Inport  Port=2
  T_r [K] : Inport  Port=3
  Constant : Constant  Value=A_c
  Constant1 : Constant  Value=1.5 .* par.Tc
  Constant3 : Constant  Value=1.5 .* par.Tc
  Divide : Product  Inputs=*/
  F0021_cp.m : base_lib/F0021_R1234yf/F0021_cp.m  SystemSampleTime=-1  VariantActivationTime=update diagram  Latency=0  AutoFrameSizeCalculation=off
      settings: LibrarySourceBlock=|
      | simulink/User-Defined
      | Functions/MATLAB Function
  F0021_cp.m1 : base_lib/F0021_R1234yf/F0021_cp.m  SystemSampleTime=-1  VariantActivationTime=update diagram  Latency=0  AutoFrameSizeCalculation=off
      settings: LibrarySourceBlock=|
      | simulink/User-Defined
      | Functions/MATLAB Function
  F0021_cv.m : base_lib/F0021_R1234yf/F0021_cv.m  SystemSampleTime=-1  VariantActivationTime=update diagram  Latency=0  AutoFrameSizeCalculation=off
      settings: LibrarySourceBlock=|
      | simulink/User-Defined
      | Functions/MATLAB Function
  F0021_cv.m1 : base_lib/F0021_R1234yf/F0021_cv.m  SystemSampleTime=-1  VariantActivationTime=update diagram  Latency=0  AutoFrameSizeCalculation=off
      settings: LibrarySourceBlock=|
      | simulink/User-Defined
      | Functions/MATLAB Function
  F0021_dliqsat.m : base_lib/F0021_R1234yf/F0021_dliqsat.m  SystemSampleTime=-1  VariantActivationTime=update diagram  Latency=0  AutoFrameSizeCalculation=off
      settings: LibrarySourceBlock=|
      | simulink/User-Defined
      | Functions/MATLAB Function
  F0021_dpdrho.m{,1..3} (4 alike) : base_lib/F0021_R1234yf/F0021_dpdrho.m  SystemSampleTime=-1  VariantActivationTime=update diagram  Latency=0  AutoFrameSizeCalculation=off
      settings: LibrarySourceBlock=|
      | simulink/User-Defined
      | Functions/MATLAB Function
  F0021_dvapsat.m : base_lib/F0021_R1234yf/F0021_dvapsat.m  SystemSampleTime=-1  VariantActivationTime=update diagram  Latency=0  AutoFrameSizeCalculation=off
      settings: LibrarySourceBlock=|
      | simulink/User-Defined
      | Functions/MATLAB Function
  F0022_OSFPHEX.m : base_lib/F0022_heatPump/F0022_OSFPHEX.m  SystemSampleTime=-1  VariantActivationTime=update diagram  Latency=0  AutoFrameSizeCalculation=off
      settings: LibrarySourceBlock=|
      | simulink/User-Defined
      | Functions/MATLAB Function
  Gain1 : Gain  Gain=1/par.M
  Gain4 : Gain  Gain=1/par.M
  Gain7 : Gain  Gain=par.M
  Gain9 : Gain  Gain=par.M
  R1234yf_lambda.m : base_lib/F0021_R1234yf/R1234yf_lambda.m  SystemSampleTime=-1  VariantActivationTime=update diagram  Latency=0  AutoFrameSizeCalculation=off
      settings: LibrarySourceBlock=|
      | simulink/User-Defined
      | Functions/MATLAB Function
  R1234yf_lambda.m1 : base_lib/F0021_R1234yf/R1234yf_lambda.m  SystemSampleTime=-1  VariantActivationTime=update diagram  Latency=0  AutoFrameSizeCalculation=off
      settings: LibrarySourceBlock=|
      | simulink/User-Defined
      | Functions/MATLAB Function
  R1234yf_mu.m : base_lib/F0021_R1234yf/R1234yf_mu.m  SystemSampleTime=-1  VariantActivationTime=update diagram  Latency=0  AutoFrameSizeCalculation=off
      settings: LibrarySourceBlock=|
      | simulink/User-Defined
      | Functions/MATLAB Function
  R1234yf_mu.m1 : base_lib/F0021_R1234yf/R1234yf_mu.m  SystemSampleTime=-1  VariantActivationTime=update diagram  Latency=0  AutoFrameSizeCalculation=off
      settings: LibrarySourceBlock=|
      | simulink/User-Defined
      | Functions/MATLAB Function
  R1234yf_sigma.m : base_lib/F0021_R1234yf/R1234yf_sigma.m  SystemSampleTime=-1  VariantActivationTime=update diagram  Latency=0  AutoFrameSizeCalculation=off
      settings: LibrarySourceBlock=|
      | simulink/User-Defined
      | Functions/MATLAB Function
  h [W/mK] : Outport
  wires:
  [cp_f] -> R1234yf_lambda.m/3
  Divide/1 -> F0022_OSFPHEX.m/1
  F0021_dpdrho.m1/1 -> R1234yf_lambda.m/7
  F0021_dliqsat.m/1 -> F0021_dpdrho.m1/2, F0021_dpdrho.m/2, F0021_cv.m/2, R1234yf_lambda.m/2, R1234yf_mu.m/2, F0021_cp.m/2, Gain9/1
  F0021_cv.m/1 -> R1234yf_lambda.m/4
  Constant3/1 -> F0021_dpdrho.m1/1
  R1234yf_mu.m/1 -> F0022_OSFPHEX.m/7, [mu_f]
  x_r [-]/1 -> F0022_OSFPHEX.m/2
  F0021_dpdrho.m/1 -> R1234yf_lambda.m/6
  R1234yf_sigma.m/1 -> F0022_OSFPHEX.m/11
  F0021_dvapsat.m/1 -> R1234yf_lambda.m1/2, F0021_dpdrho.m3/2, F0021_dpdrho.m2/2, F0021_cv.m1/2, R1234yf_mu.m1/2, F0021_cp.m1/2, Gain7/1
  Gain7/1 -> F0022_OSFPHEX.m/4
  R1234yf_lambda.m/1 -> F0022_OSFPHEX.m/9
  [mu_f] -> R1234yf_lambda.m/5
  W_r [kg/s]/1 -> Divide/1
  Gain4/1 -> F0022_OSFPHEX.m/5
  Gain9/1 -> F0022_OSFPHEX.m/3
  F0021_cp.m/1 -> [cp_f], Gain4/1
  F0022_OSFPHEX.m/1 -> h [W/mK]/1
  Gain1/1 -> F0022_OSFPHEX.m/6
  F0021_cp.m1/1 -> [cp_g], Gain1/1
  R1234yf_mu.m1/1 -> [mu_g], F0022_OSFPHEX.m/8
  [mu_g] -> R1234yf_lambda.m1/5
  Constant1/1 -> F0021_dpdrho.m3/1
  T_r [K]/1 -> F0021_cp.m1/1, R1234yf_mu.m1/1, F0021_dpdrho.m2/1, F0021_cv.m1/1, R1234yf_lambda.m1/1, F0021_dpdrho.m/1, F0021_cv.m/1, R1234yf_lambda.m/1, R1234yf_sigma.m/1, R1234yf_mu.m/1, F0021_cp.m/1, F0021_dvapsat.m/1, F0021_dliqsat.m/1
  F0021_dpdrho.m3/1 -> R1234yf_lambda.m1/7
  F0021_cv.m1/1 -> R1234yf_lambda.m1/4
  F0021_dpdrho.m2/1 -> R1234yf_lambda.m1/6
  [cp_g] -> R1234yf_lambda.m1/3
  R1234yf_lambda.m1/1 -> F0022_OSFPHEX.m/10
  Constant/1 -> Divide/2

== system component_lib/Thermal Systems/RF0012_louverFinHEX/Heat Tranfer Coefficient - Refrigerant Side ==
  W_r [kg/s] : Inport
  x_r [-] : Inport  Port=2
  T_r [K] : Inport  Port=3
  Abs : Abs  SaturateOnIntegerOverflow=off
  Constant1 : Constant  Value=1.5 .* par.Tc
  Constant3 : Constant  Value=1.5 .* par.Tc
  F0021_cp.m : base_lib/F0021_R1234yf/F0021_cp.m  SystemSampleTime=-1  VariantActivationTime=update diagram  Latency=0  AutoFrameSizeCalculation=off
      settings: LibrarySourceBlock=|
      | simulink/User-Defined
      | Functions/MATLAB Function
  F0021_cp.m1 : base_lib/F0021_R1234yf/F0021_cp.m  SystemSampleTime=-1  VariantActivationTime=update diagram  Latency=0  AutoFrameSizeCalculation=off
      settings: LibrarySourceBlock=|
      | simulink/User-Defined
      | Functions/MATLAB Function
  F0021_cv.m : base_lib/F0021_R1234yf/F0021_cv.m  SystemSampleTime=-1  VariantActivationTime=update diagram  Latency=0  AutoFrameSizeCalculation=off
      settings: LibrarySourceBlock=|
      | simulink/User-Defined
      | Functions/MATLAB Function
  F0021_cv.m1 : base_lib/F0021_R1234yf/F0021_cv.m  SystemSampleTime=-1  VariantActivationTime=update diagram  Latency=0  AutoFrameSizeCalculation=off
      settings: LibrarySourceBlock=|
      | simulink/User-Defined
      | Functions/MATLAB Function
  F0021_dliqsat.m : base_lib/F0021_R1234yf/F0021_dliqsat.m  SystemSampleTime=-1  VariantActivationTime=update diagram  Latency=0  AutoFrameSizeCalculation=off
      settings: LibrarySourceBlock=|
      | simulink/User-Defined
      | Functions/MATLAB Function
  F0021_dpdrho.m{,1..3} (4 alike) : base_lib/F0021_R1234yf/F0021_dpdrho.m  SystemSampleTime=-1  VariantActivationTime=update diagram  Latency=0  AutoFrameSizeCalculation=off
      settings: LibrarySourceBlock=|
      | simulink/User-Defined
      | Functions/MATLAB Function
  F0021_dvapsat.m : base_lib/F0021_R1234yf/F0021_dvapsat.m  SystemSampleTime=-1  VariantActivationTime=update diagram  Latency=0  AutoFrameSizeCalculation=off
      settings: LibrarySourceBlock=|
      | simulink/User-Defined
      | Functions/MATLAB Function
  F0021_psat.m : base_lib/F0021_R1234yf/F0021_psat.m  SystemSampleTime=-1  VariantActivationTime=update diagram  Latency=0  AutoFrameSizeCalculation=off
      settings: LibrarySourceBlock=|
      | simulink/User-Defined
      | Functions/MATLAB Function
  F0022_massFlux.m : base_lib/F0022_heatPump/F0022_massFlux.m  SystemSampleTime=-1  VariantActivationTime=update diagram  Latency=0  AutoFrameSizeCalculation=off
      settings: LibrarySourceBlock=|
      | simulink/User-Defined
      | Functions/MATLAB Function
  F0022_minichannelCondensingHTC.m : base_lib/F0022_heatPump/F0022_minichannelCondensingHTC.m  SystemSampleTime=-1  VariantActivationTime=update diagram  Latency=0  AutoFrameSizeCalculation=off
      settings: LibrarySourceBlock=|
      | simulink/User-Defined
      | Functions/MATLAB Function
  Gain1 : Gain  Gain=1/par.M
  Gain4 : Gain  Gain=1/par.M
  Gain7 : Gain  Gain=par.M
  Gain9 : Gain  Gain=par.M
  R1234yf_lambda.m : base_lib/F0021_R1234yf/R1234yf_lambda.m  SystemSampleTime=-1  VariantActivationTime=update diagram  Latency=0  AutoFrameSizeCalculation=off
      settings: LibrarySourceBlock=|
      | simulink/User-Defined
      | Functions/MATLAB Function
  R1234yf_lambda.m1 : base_lib/F0021_R1234yf/R1234yf_lambda.m  SystemSampleTime=-1  VariantActivationTime=update diagram  Latency=0  AutoFrameSizeCalculation=off
      settings: LibrarySourceBlock=|
      | simulink/User-Defined
      | Functions/MATLAB Function
  R1234yf_mu.m : base_lib/F0021_R1234yf/R1234yf_mu.m  SystemSampleTime=-1  VariantActivationTime=update diagram  Latency=0  AutoFrameSizeCalculation=off
      settings: LibrarySourceBlock=|
      | simulink/User-Defined
      | Functions/MATLAB Function
  R1234yf_mu.m1 : base_lib/F0021_R1234yf/R1234yf_mu.m  SystemSampleTime=-1  VariantActivationTime=update diagram  Latency=0  AutoFrameSizeCalculation=off
      settings: LibrarySourceBlock=|
      | simulink/User-Defined
      | Functions/MATLAB Function
  h [W/mK] : Outport
  wires:
  F0022_minichannelCondensingHTC.m/1 -> h [W/mK]/1
  W_r [kg/s]/1 -> Abs/1
  F0021_cp.m/1 -> [cp_f], Gain4/1
  Gain9/1 -> F0022_minichannelCondensingHTC.m/4
  Gain4/1 -> F0022_minichannelCondensingHTC.m/6
  Abs/1 -> F0022_massFlux.m/1
  [mu_f] -> R1234yf_lambda.m/5
  F0021_dvapsat.m/1 -> [rho_g], Gain7/1, F0021_cp.m1/2, R1234yf_mu.m1/2
  F0021_dpdrho.m/1 -> R1234yf_lambda.m/6
  R1234yf_mu.m/1 -> F0022_minichannelCondensingHTC.m/8, [mu_f]
  Constant3/1 -> F0021_dpdrho.m1/1
  F0021_cv.m/1 -> R1234yf_lambda.m/4
  F0021_dliqsat.m/1 -> R1234yf_mu.m/2, F0021_cp.m/2, [rho_f], Gain9/1
  F0021_dpdrho.m1/1 -> R1234yf_lambda.m/7
  F0022_massFlux.m/1 -> F0022_minichannelCondensingHTC.m/1
  [cp_f] -> R1234yf_lambda.m/3
  Gain7/1 -> F0022_minichannelCondensingHTC.m/5
  [rho_f] -> F0021_dpdrho.m1/2, F0021_dpdrho.m/2, F0021_cv.m/2, R1234yf_lambda.m/2
  F0021_psat.m/1 -> F0022_minichannelCondensingHTC.m/2
  F0021_cp.m1/1 -> [cp_g], Gain1/1
  Gain1/1 -> F0022_minichannelCondensingHTC.m/7
  R1234yf_mu.m1/1 -> [mu_g], F0022_minichannelCondensingHTC.m/9
  [rho_g] -> F0021_dpdrho.m3/2, F0021_dpdrho.m2/2, F0021_cv.m1/2, R1234yf_lambda.m1/2
  [cp_g] -> R1234yf_lambda.m1/3
  F0021_dpdrho.m3/1 -> R1234yf_lambda.m1/7
  Constant1/1 -> F0021_dpdrho.m3/1
  [mu_g] -> R1234yf_lambda.m1/5
  T_r [K]/1 -> F0021_cp.m1/1, R1234yf_mu.m/1, F0021_dpdrho.m2/1, F0021_cv.m1/1, R1234yf_lambda.m1/1, F0021_dpdrho.m/1, F0021_cv.m/1, R1234yf_lambda.m/1, R1234yf_mu.m1/1, F0021_cp.m/1, F0021_dvapsat.m/1, F0021_dliqsat.m/1, F0021_psat.m/1
  F0021_dpdrho.m2/1 -> R1234yf_lambda.m1/6
  F0021_cv.m1/1 -> R1234yf_lambda.m1/4
  R1234yf_lambda.m1/1 -> F0022_minichannelCondensingHTC.m/11
  R1234yf_lambda.m/1 -> F0022_minichannelCondensingHTC.m/10
  x_r [-]/1 -> F0022_minichannelCondensingHTC.m/3

== matlab function component_lib/Data & Control/DC0008_linearMPCSolver/MPCtoQP ==
  data: A input; B input; Q input; R input; N input; P output; c output; A_eq output; b output; G output; h output
function [P,c,A_eq,b,G,h] = MPCtoQP(A,B,Q,R,N)

% Q_bar = blkdiag( 
% R_bar = 



% outputs
P    = [];
c    =  [];
A_eq = [];
b    = [];
G    = [];
h    = [];


% output in column major format
P = P(:);
K = K(:);
G = G(:);
